simulink model "Relay_Feedback_Method"  (R2023a)
settings: Solver=VariableStepAuto  StartTime=0.0  StopTime=200  RelTol=1e-3
values from neighbouring files (symbols this model uses):
  A_alpha = -.1    (= -0.1)    [main.m]
  A_beta = 10    [main.m]
  A_wind = -1    [main.m]
  bool_alpha = 0    [main.m]
  bool_beta = 0    [main.m]
  bool_wind = 0    [main.m]
  G_D_sim = table_tf(table_tf.wind_speed==v_wind,:).G_D    [main.m]
  G_S_sim = table_tf(table_tf.wind_speed==v_wind,:).G_S    [main.m]
  pulse_width = 50    [main.m]
  T_delay = 600    [main.m]
  T_period = 1200    [main.m]
libraries: cstblocks x2
settings Model: Creator=pascalbock  LastModifiedBy=pascalbock

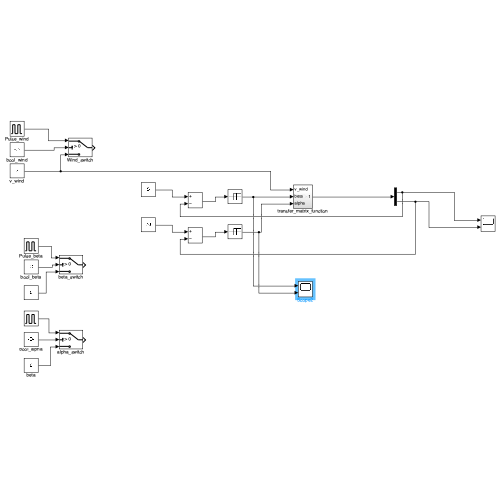
[thumbnail: Simulink's stored preview of the top-level diagram]
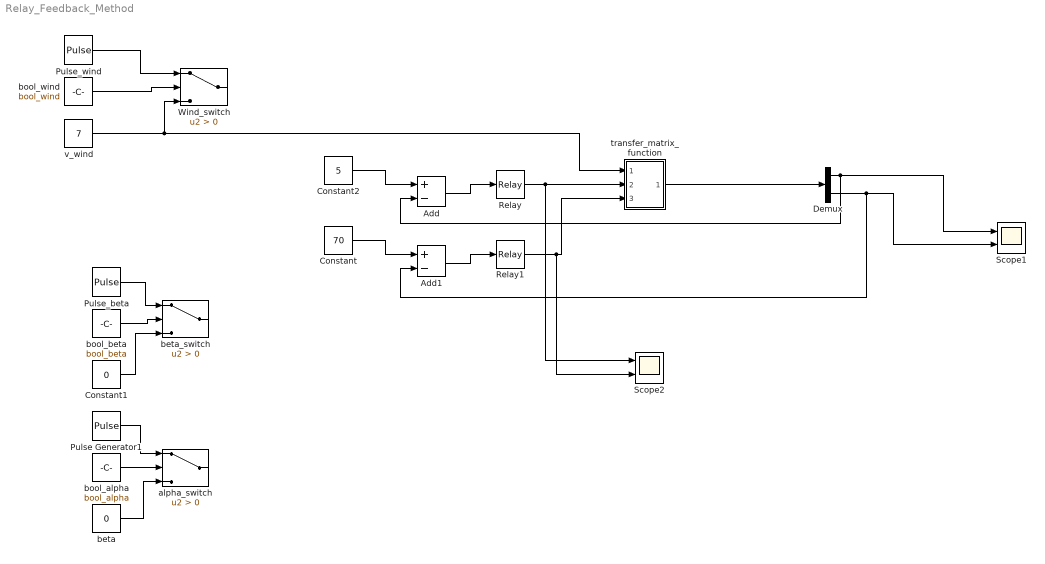
== system Relay_Feedback_Method ==
  Add : Sum  Inputs=+-
  Add1 : Sum  Inputs=+-
  Constant : Constant  Value=70
  Constant1 : Constant  Value=0
  Constant2 : Constant  Value=5
  Demux : Demux  Outputs=2
  Pulse Generator1 : DiscretePulseGenerator  PulseType=Time based  Amplitude=A_alpha  Period=T_period  PulseWidth=pulse_width  PhaseDelay=T_delay
  Pulse_beta : DiscretePulseGenerator  PulseType=Time based  Amplitude=A_beta  Period=T_period  PulseWidth=pulse_width  PhaseDelay=T_delay
  Pulse_wind : DiscretePulseGenerator  PulseType=Time based  Amplitude=A_wind  Period=T_period  PulseWidth=pulse_width  PhaseDelay=T_delay
  Relay : Relay  OnSwitchValue=5*1.03  OffSwitchValue=5*0.97  OnOutputValue=0  OffOutputValue=1
  Relay1 : Relay  OnSwitchValue=70*1.03  OffSwitchValue=70*0.97  OnOutputValue=5
  Scope1 : Scope  NumInputPorts=2
  Scope2 : Scope  NumInputPorts=2
  Wind_switch : Switch  Criteria=u2 > Threshold  SaturateOnIntegerOverflow=off  InputSameDT=off
  alpha_switch : Switch  Criteria=u2 > Threshold  SaturateOnIntegerOverflow=off  InputSameDT=off
  beta : Constant  Value=0
  beta_switch : Switch  Criteria=u2 > Threshold  SaturateOnIntegerOverflow=off  InputSameDT=off
  bool_alpha : Constant  Value=bool_alpha
  bool_beta : Constant  Value=bool_beta
  bool_wind : Constant  Value=bool_wind
  transfer_matrix_function : Subsystem
  v_wind : Constant  Value=7
  wires:
  transfer_matrix_function/1(Out1) -> Demux/1
  Demux/1 -> Add/2, Scope1/1
  Pulse_wind/1 -> Wind_switch/1
  v_wind/1 -> transfer_matrix_function/1(v_wind), Wind_switch/3
  bool_wind/1 -> Wind_switch/2
  bool_alpha/1 -> alpha_switch/2
  beta/1 -> alpha_switch/3
  Pulse_beta/1 -> beta_switch/1
  Pulse Generator1/1 -> alpha_switch/1
  bool_beta/1 -> beta_switch/2
  Constant1/1 -> beta_switch/3
  Constant2/1 -> Add/1
  Add/1 -> Relay/1
  Relay/1 -> Scope2/1, transfer_matrix_function/2(beta)
  Demux/2 -> Add1/2, Scope1/2
  Add1/1 -> Relay1/1
  Constant/1 -> Add1/1
  Relay1/1 -> Scope2/2, transfer_matrix_function/3(alpha)

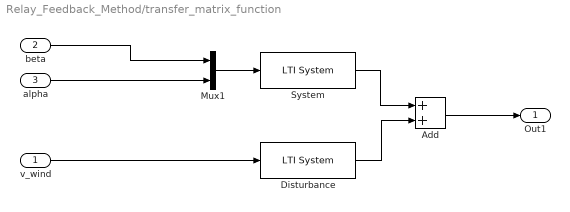
== system Relay_Feedback_Method/transfer_matrix_function ==
  v_wind : Inport
  beta : Inport  Port=2
  alpha : Inport  Port=3
  Add : Sum
  Disturbance : cstblocks/LTI System  sys=G_D_sim{1}  IC=[]
  Mux1 : Mux  Inputs=2
  System : cstblocks/LTI System  sys=G_S_sim{1}  IC=[]
  Out1 : Outport
  wires:
  Add/1 -> Out1/1
  Disturbance/1 -> Add/2
  System/1 -> Add/1
  Mux1/1 -> System/1
  alpha/1 -> Mux1/2
  v_wind/1 -> Disturbance/1
  beta/1 -> Mux1/1
